simulink model "V2x_TC_CarBreakdownWarning_cs"  (Simulink 7.6)
settings: Solver=ode5  SolverMode=SingleTasking  StartTime=0.0  StopTime=18  FixedStep=1/100  RelTol=1e-3
PreLoadFcn:
  | check_NUTS_defined;
  | 
  | assignin('base',['model_closed_' bdroot],false);addpath('../includes_V2x');
InitFcn:
  | PreScanExperimentInitFcn(bdroot)
StopFcn:
  | PreScanExperimentStopFcn(bdroot)
undefined symbols (not defined in the file or in its folder): acceleration, actorID, actorType, DiscIntNeverNeededParam, GPS_alt, GPS_lat, GPS_long, intmax, lightBarInUse, messageID, Newton, publicActorType, Raphson, rotZ, sigbuilder_block, sireneInUse, trafficLightPriority, turnAdvice, velocity, x_ini_VRML, y_ini_VRML, yawRate, z_ini_VRML
libraries: simulink x61, PreScanSimulinkLibrary x19, PreScanUsefulBlocks x7, simulink_extras x1
(part 8 of 10)

== system V2x_TC_CarBreakdownWarning_cs/BMW_X5_1/Trajectories/Traj2State1 ==
  Traj Org : Inport
  Offset : Inport  Port=2
  Add2 : Sum
  ApplyRotation : PreScanSimulinkLibrary/ApplyRotation  SystemSampleTime=-1
  ApplyRotation1 : PreScanSimulinkLibrary/ApplyRotation  SystemSampleTime=-1
  ApplyRotation2 : PreScanSimulinkLibrary/ApplyRotation  SystemSampleTime=-1
  Constant : Constant  Value=zeros(12,1)
  Mux : Mux  Inputs=6
  Mux1 : Mux  Inputs=2
  Mux{2,4..9} (7 alike) : Mux  Inputs=3
  Mux3 : Mux  Inputs=2
  Selector : Selector  InputPortWidth=6  IndexOptions=Index vector (dialog)  Indices=[4 5 6]  OutputSizes=1
  Selector1 : Selector  InputPortWidth=21  IndexOptions=Index vector (dialog)  Indices=[5]  OutputSizes=1
  Selector10 : Selector  InputPortWidth=21  IndexOptions=Index vector (dialog)  Indices=[2]  OutputSizes=1
  Selector11 : Selector  InputPortWidth=21  IndexOptions=Index vector (dialog)  Indices=[3]  OutputSizes=1
  Selector12 : Selector  InputPortWidth=21  IndexOptions=Index vector (dialog)  Indices=[1]  OutputSizes=1
  Selector13 : Selector  InputPortWidth=21  IndexOptions=Index vector (dialog)  Indices=[8]  OutputSizes=1
  Selector14 : Selector  InputPortWidth=21  IndexOptions=Index vector (dialog)  Indices=[9]  OutputSizes=1
  Selector15 : Selector  InputPortWidth=21  IndexOptions=Index vector (dialog)  Indices=[7]  OutputSizes=1
  Selector16 : Selector  InputPortWidth=21  IndexOptions=Index vector (dialog)  Indices=[14]  OutputSizes=1
  Selector17 : Selector  InputPortWidth=21  IndexOptions=Index vector (dialog)  Indices=[15]  OutputSizes=1
  Selector18 : Selector  InputPortWidth=21  IndexOptions=Index vector (dialog)  Indices=[13]  OutputSizes=1
  Selector19 : Selector  InputPortWidth=21  IndexOptions=Index vector (dialog)  Indices=[20]  OutputSizes=1
  Selector2 : Selector  InputPortWidth=21  IndexOptions=Index vector (dialog)  Indices=[6]  OutputSizes=1
  Selector20 : Selector  InputPortWidth=21  IndexOptions=Index vector (dialog)  Indices=[21]  OutputSizes=1
  Selector21 : Selector  InputPortWidth=21  IndexOptions=Index vector (dialog)  Indices=[19]  OutputSizes=1
  Selector3 : Selector  InputPortWidth=21  IndexOptions=Index vector (dialog)  Indices=[12]  OutputSizes=1
  Selector4 : Selector  InputPortWidth=21  IndexOptions=Index vector (dialog)  Indices=[17]  OutputSizes=1
  Selector5 : Selector  InputPortWidth=21  IndexOptions=Index vector (dialog)  Indices=[18]  OutputSizes=1
  Selector6 : Selector  InputPortWidth=21  IndexOptions=Index vector (dialog)  Indices=[16]  OutputSizes=1
  Selector7 : Selector  InputPortWidth=21  IndexOptions=Index vector (dialog)  Indices=[11]  OutputSizes=1
  Selector8 : Selector  InputPortWidth=21  IndexOptions=Index vector (dialog)  Indices=[10]  OutputSizes=1
  Selector9 : Selector  InputPortWidth=21  IndexOptions=Index vector (dialog)  Indices=[4]  OutputSizes=1
  Traj2State2 : Subsystem
  state : Outport
  wires:
  Mux9/1 -> ApplyRotation2/2, ApplyRotation1/2, ApplyRotation/2
  Selector20/1 -> Mux9/3
  Selector19/1 -> Mux9/2
  Selector21/1 -> Mux9/1
  Selector5/1 -> Mux8/3
  Selector4/1 -> Mux8/2
  Selector6/1 -> Mux8/1
  Mux8/1 -> Mux/6
  Mux6/1 -> ApplyRotation2/1
  Mux7/1 -> Mux/4
  ApplyRotation2/1 -> Mux/5
  Selector3/1 -> Mux7/3
  Selector7/1 -> Mux7/2
  Selector8/1 -> Mux7/1
  Mux4/1 -> Mux/2
  Mux5/1 -> ApplyRotation1/1
  ApplyRotation1/1 -> Mux/3
  Mux2/1 -> ApplyRotation/1
  ApplyRotation/1 -> Mux/1
  Selector2/1 -> Mux4/3
  Selector1/1 -> Mux4/2
  Selector9/1 -> Mux4/1
  Selector17/1 -> Mux6/3
  Selector16/1 -> Mux6/2
  Selector18/1 -> Mux6/1
  Selector14/1 -> Mux5/3
  Selector13/1 -> Mux5/2
  Selector15/1 -> Mux5/1
  Selector11/1 -> Mux2/3
  Selector10/1 -> Mux2/2
  Selector12/1 -> Mux2/1
  Mux3/1 -> Selector8/1, Selector7/1, Selector3/1, Selector18/1, Selector16/1, Selector17/1, Selector6/1, Selector20/1, Selector19/1, Selector21/1, Selector5/1, Selector4/1, Selector14/1, Selector13/1, Selector15/1, Selector2/1, Selector1/1, Selector9/1, Selector12/1, Selector10/1, Selector11/1
  Mux1/1 -> Add2/2
  Constant/1 -> Mux1/2
  Add2/1 -> Traj2State2/1(traj)
  Selector/1 -> Mux3/2
  Traj Org/1 -> Mux3/1
  Offset/1 -> Mux1/1, Selector/1
  Mux/1 -> Add2/1
  Traj2State2/1(state) -> state/1

== system V2x_TC_CarBreakdownWarning_cs/BMW_X5_1/Trajectories/Trajectory_4 ==
  From Workspace : FromWorkspace  VariableName=trajectory  SampleTime=TimeStep  OutputAfterFinalValue=Holding final value
  From Workspace1 : FromWorkspace  VariableName=trajectory  SampleTime=TimeStep  OutputAfterFinalValue=Setting to zero
  Mux : Mux  Inputs=2
  Selector1 : Selector  InputPortWidth=24  IndexOptions=Index vector (dialog)  Indices=[7:18]  OutputSizes=1
  Selector9 : Selector  InputPortWidth=24  IndexOptions=Index vector (dialog)  Indices=[1:6]  OutputSizes=1
  trajectory : Outport
  wires:
  Selector1/1 -> Mux/2
  Selector9/1 -> Mux/1
  Mux/1 -> trajectory/1
  From Workspace1/1 -> Selector1/1
  From Workspace/1 -> Selector9/1

== system V2x_TC_CarBreakdownWarning_cs/BMW_X5_1/vehicle CAM generator/CAM generation ==
  x [m] : Inport
  y [m] : Inport  Port=2
  z [m] : Inport  Port=3
  rotZ [deg] : Inport  Port=4
  velocity [m/s] : Inport  Port=5
  Enable : EnablePort  StatesWhenEnabling=reset  PropagateVarSize=During execution
  Add : Sum  Inputs=+-
  Data Store Memory : DataStoreMemory  DataStoreName=CAM_time
  Data Store Memory1 : DataStoreMemory  DataStoreName=CAM_velocity
  Data Store Memory2 : DataStoreMemory  DataStoreName=CAM_heading
  Data Store Memory3 : DataStoreMemory  DataStoreName=CAM_x
  Data Store Memory4 : DataStoreMemory  DataStoreName=CAM_y
  Data Store Memory5 : DataStoreMemory  DataStoreName=CAM_z
  Data Store Read : DataStoreRead  DataStoreName=CAM_time  SampleTime=0.01
  Digital Clock : DigitalClock  SampleTime=0.01
  Merge : Merge  Inputs=3
  if : If  IfExpression=u1 >= 1  ElseIfExpressions=u1 < 0.1
  maybe : Subsystem  TreatAsAtomicUnit=on
  no : Subsystem  TreatAsAtomicUnit=on
  yes : Subsystem  TreatAsAtomicUnit=on
  CAN generation signal : Outport  OutputWhenDisabled=reset  InitialOutput=0
  wires:
  Digital Clock/1 -> Add/1
  Data Store Read/1 -> Add/2
  Add/1 -> if/1
  if/1 -> yes/Action
  yes/1(Out1) -> Merge/1
  no/1(Out1) -> Merge/2
  if/2 -> no/Action
  if/3 -> maybe/Action
  Merge/1 -> CAN generation signal/1
  x [m]/1 -> maybe/1(x [m]), yes/1(x [m])
  y [m]/1 -> maybe/2(y [m]), yes/2(y [m])
  z [m]/1 -> maybe/3(z [m]), yes/3(z [m])
  rotZ [deg]/1 -> maybe/4(rotZ [deg]), yes/4(rotZ [deg])
  velocity [m/s]/1 -> maybe/5(velocity [m/s]), yes/5(velocity [m/s])
  maybe/1(Out1) -> Merge/3

== system V2x_TC_CarBreakdownWarning_cs/BMW_X5_1/vehicle CAM generator/Enabled Subsystem ==
  CAM_sig : Inport
  Enable : EnablePort  PropagateVarSize=During execution
  CAM_signals : Outport  OutputWhenDisabled=reset  InitialOutput=0
  wires:
  CAM_sig/1 -> CAM_signals/1

== system V2x_TC_CarBreakdownWarning_cs/BMW_X5_1/vehicle CAM generator/impulse generator ==
  CAM_time_step : Inport
  Add : Sum
  Compare To Zero : simulink/Logic and Bit Operations/Compare To Zero  SystemSampleTime=-1  relop=>  LogicOutDataTypeMode=uint8  ZeroCross=off
  Data Type Conversion : DataTypeConversion  OutDataTypeStr=boolean
  Detect Change : simulink/Logic and Bit Operations/Detect Change  SystemSampleTime=-1  vinit=0
  Digital Clock1 : DigitalClock  SampleTime=0.01
  Divide : Product  Inputs=*/
  Gain : Gain  Gain=pi
  Product : Product  RndMeth=Zero
  Trigonometric Function : Trigonometry
  constant : Constant
  experiment time step : Constant  Value=0.01  SampleTime=0
  enable : Outport
  wires:
  Digital Clock1/1 -> Product/1
  Gain/1 -> Product/2
  Trigonometric Function/1 -> Compare To Zero/1
  Compare To Zero/1 -> Detect Change/1
  Detect Change/1 -> Data Type Conversion/1
  Product/1 -> Add/1
  constant/1 -> Divide/1
  Divide/1 -> Gain/1
  Add/1 -> Trigonometric Function/1
  experiment time step/1 -> Add/2
  Data Type Conversion/1 -> enable/1
  CAM_time_step/1 -> Divide/2

== system V2x_TC_CarBreakdownWarning_cs/BMW_X5_1/vehicle CAM generator/impulse generator1 ==
  CAM_time_step : Inport
  Add : Sum
  Compare To Zero : simulink/Logic and Bit Operations/Compare To Zero  SystemSampleTime=-1  relop=>  LogicOutDataTypeMode=uint8  ZeroCross=off
  Data Type Conversion : DataTypeConversion  OutDataTypeStr=boolean
  Detect Change : simulink/Logic and Bit Operations/Detect Change  SystemSampleTime=-1  vinit=0
  Digital Clock1 : DigitalClock  SampleTime=0.01
  Divide : Product  Inputs=*/
  Gain : Gain  Gain=pi
  Product : Product  RndMeth=Zero
  Trigonometric Function : Trigonometry
  constant : Constant
  experiment time step : Constant  Value=0.01  SampleTime=0
  enable : Outport
  wires:
  CAM_time_step/1 -> Divide/2
  Data Type Conversion/1 -> enable/1
  experiment time step/1 -> Add/2
  Add/1 -> Trigonometric Function/1
  Divide/1 -> Gain/1
  constant/1 -> Divide/1
  Product/1 -> Add/1
  Detect Change/1 -> Data Type Conversion/1
  Compare To Zero/1 -> Detect Change/1
  Trigonometric Function/1 -> Compare To Zero/1
  Gain/1 -> Product/2
  Digital Clock1/1 -> Product/1

== system V2x_TC_CarBreakdownWarning_cs/BMW_X5_1/vehicle CAM generator/set CAM signals ==
  CAM generation signal : Inport
  warning : Inport  Port=2
  messageID : Inport  Port=3
  actorID : Inport  Port=4
  actorType : Inport  Port=5
  publicActorType : Inport  Port=6
  lightBarInUse : Inport  Port=7
  sireneInUse : Inport  Port=8
  velocity : Inport  Port=9
  acceleration : Inport  Port=10
  yawRate : Inport  Port=11
  turnAdvice : Inport  Port=12
  trafficLightPriority : Inport  Port=13
  GPS_lat : Inport  Port=14
  GPS_long : Inport  Port=15
  GPS_alt : Inport  Port=16
  rotZ : Inport  Port=17
  Mux : Mux  Inputs=16
  Switch : Switch  Criteria=u2 > Threshold  Threshold=0.5
  Unit Delay : UnitDelay  SampleTime=-1
  CAM_signals : Outport
  wires:
  warning/1 -> Mux/1
  messageID/1 -> Mux/2
  actorID/1 -> Mux/3
  actorType/1 -> Mux/4
  publicActorType/1 -> Mux/5
  lightBarInUse/1 -> Mux/6
  sireneInUse/1 -> Mux/7
  velocity/1 -> Mux/8
  acceleration/1 -> Mux/9
  yawRate/1 -> Mux/10
  turnAdvice/1 -> Mux/11
  trafficLightPriority/1 -> Mux/12
  GPS_lat/1 -> Mux/13
  GPS_long/1 -> Mux/14
  GPS_alt/1 -> Mux/15
  rotZ/1 -> Mux/16
  CAM generation signal/1 -> Switch/2
  Mux/1 -> Switch/1
  Switch/1 -> Unit Delay/1, CAM_signals/1
  Unit Delay/1 -> Switch/3

== system V2x_TC_CarBreakdownWarning_cs/CameraTrolley/Dynamics_Empty/MuxState ==
  note: mode: Dynamics
  note: mode: Positioning
  note: mode: Dynamics
      | VelVEHICLE
      | wrt VEH
  note: AnglesVEHICLE
      | wrtGLOB
  note: For state mode 'Dynamic' positions
      | are not taken into account, as they
      | are computed by integrating velocity.
      | Click annotation for Help.
  x [m] : Inport  SampleTime=TimeStep
  y [m] : Inport  Port=2  SampleTime=TimeStep
  z [m] : Inport  Port=3  SampleTime=TimeStep
  dx [m/s] : Inport  Port=4  SampleTime=TimeStep
  dy [m/s] : Inport  Port=5  SampleTime=TimeStep
  dz [m/s] : Inport  Port=6  SampleTime=TimeStep
  R [rad] : Inport  Port=7  SampleTime=TimeStep
  P [rad] : Inport  Port=8  SampleTime=TimeStep
  Y [rad] : Inport  Port=9  SampleTime=TimeStep
  Constant : Constant  DisableCoverage=on  Value=positioningmode
  Discrete-Time Integrator : DiscreteIntegrator  SampleTime=TimeStep  ICPrevOutput=DiscIntNeverNeededParam  ICPrevScaledInput=DiscIntNeverNeededParam
  Ground : Ground
  Ground1 : Ground
  Mux1 : Mux  Inputs=[3 3]
  Mux2 : Mux  Inputs=3
  Mux3 : Mux  Inputs=3
  Mux4 : Mux  Inputs=3
  Mux5 : Mux  Inputs=[3 3]
  Mux6 : Mux  Inputs=[6 3]
  Switch : Switch  Threshold=0.5
  Transformation_BODY2GLOBAL : PreScanSimulinkLibrary/Simple_Vehicle_Dynamics/Chassis/MuxDynState/Transformation_BODY2GLOBAL  SystemSampleTime=-1
  mux3 : Mux  Inputs=3
  state : Outport
  wires:
  Constant/1 -> Switch/2
  Mux6/1 -> state/1
  Mux4/1 -> Mux1/1
  Mux5/1 -> Switch/3
  Mux1/1 -> Switch/1
  Switch/1 -> Mux6/1  "PosVeh wrt  GLOB"
  P [rad]/1 -> Mux3/2
  R [rad]/1 -> Mux3/1
  dz [m/s]/1 -> Mux2/3
  dy [m/s]/1 -> Mux2/2
  dx [m/s]/1 -> Mux2/1
  z [m]/1 -> Mux4/3
  y [m]/1 -> Mux4/2
  x [m]/1 -> Mux4/1
  Ground1/1 -> mux3/2  "pitch"
  Y [rad]/1 -> mux3/3, Mux3/3  "yaw"
  Mux3/1 -> Mux6/2
  Transformation_BODY2GLOBAL/1 -> Discrete-Time Integrator/1, Mux5/2  "VelVEH wrt  GLOB"
  mux3/1 -> Transformation_BODY2GLOBAL/2
  Ground/1 -> mux3/1  "roll"
  Mux2/1 -> Mux1/2, Transformation_BODY2GLOBAL/1
  Discrete-Time Integrator/1 -> Mux5/1  "PosVEH wrt  GLOB"

== system V2x_TC_CarBreakdownWarning_cs/CameraTrolley/SELF_Demux/compas converter ==
  rotz [rad] : Inport
  cart2compas : Subsystem
  rad2deg : Gain  Gain=180/pi
  heading [deg] : Outport
  wires:
  cart2compas/1(heading [deg]) -> heading [deg]/1
  rotz [rad]/1 -> rad2deg/1
  rad2deg/1 -> cart2compas/1(Angle [deg])

== system V2x_TC_CarBreakdownWarning_cs/Fiat_Bravo_1/SELF_Demux/compas converter ==
  rotz [rad] : Inport
  cart2compas : Subsystem
  rad2deg : Gain  Gain=180/pi
  heading [deg] : Outport
  wires:
  cart2compas/1(heading [deg]) -> heading [deg]/1
  rotz [rad]/1 -> rad2deg/1
  rad2deg/1 -> cart2compas/1(Angle [deg])

== system V2x_TC_CarBreakdownWarning_cs/Fiat_Bravo_1/Trajectories/Traj2State1 ==
  Traj Org : Inport
  Offset : Inport  Port=2
  Add2 : Sum
  ApplyRotation : PreScanSimulinkLibrary/ApplyRotation  SystemSampleTime=-1
  ApplyRotation1 : PreScanSimulinkLibrary/ApplyRotation  SystemSampleTime=-1
  ApplyRotation2 : PreScanSimulinkLibrary/ApplyRotation  SystemSampleTime=-1
  Constant : Constant  Value=zeros(12,1)
  Mux : Mux  Inputs=6
  Mux1 : Mux  Inputs=2
  Mux{2,4..9} (7 alike) : Mux  Inputs=3
  Mux3 : Mux  Inputs=2
  Selector : Selector  InputPortWidth=6  IndexOptions=Index vector (dialog)  Indices=[4 5 6]  OutputSizes=1
  Selector1 : Selector  InputPortWidth=21  IndexOptions=Index vector (dialog)  Indices=[5]  OutputSizes=1
  Selector10 : Selector  InputPortWidth=21  IndexOptions=Index vector (dialog)  Indices=[2]  OutputSizes=1
  Selector11 : Selector  InputPortWidth=21  IndexOptions=Index vector (dialog)  Indices=[3]  OutputSizes=1
  Selector12 : Selector  InputPortWidth=21  IndexOptions=Index vector (dialog)  Indices=[1]  OutputSizes=1
  Selector13 : Selector  InputPortWidth=21  IndexOptions=Index vector (dialog)  Indices=[8]  OutputSizes=1
  Selector14 : Selector  InputPortWidth=21  IndexOptions=Index vector (dialog)  Indices=[9]  OutputSizes=1
  Selector15 : Selector  InputPortWidth=21  IndexOptions=Index vector (dialog)  Indices=[7]  OutputSizes=1
  Selector16 : Selector  InputPortWidth=21  IndexOptions=Index vector (dialog)  Indices=[14]  OutputSizes=1
  Selector17 : Selector  InputPortWidth=21  IndexOptions=Index vector (dialog)  Indices=[15]  OutputSizes=1
  Selector18 : Selector  InputPortWidth=21  IndexOptions=Index vector (dialog)  Indices=[13]  OutputSizes=1
  Selector19 : Selector  InputPortWidth=21  IndexOptions=Index vector (dialog)  Indices=[20]  OutputSizes=1
  Selector2 : Selector  InputPortWidth=21  IndexOptions=Index vector (dialog)  Indices=[6]  OutputSizes=1
  Selector20 : Selector  InputPortWidth=21  IndexOptions=Index vector (dialog)  Indices=[21]  OutputSizes=1
  Selector21 : Selector  InputPortWidth=21  IndexOptions=Index vector (dialog)  Indices=[19]  OutputSizes=1
  Selector3 : Selector  InputPortWidth=21  IndexOptions=Index vector (dialog)  Indices=[12]  OutputSizes=1
  Selector4 : Selector  InputPortWidth=21  IndexOptions=Index vector (dialog)  Indices=[17]  OutputSizes=1
  Selector5 : Selector  InputPortWidth=21  IndexOptions=Index vector (dialog)  Indices=[18]  OutputSizes=1
  Selector6 : Selector  InputPortWidth=21  IndexOptions=Index vector (dialog)  Indices=[16]  OutputSizes=1
  Selector7 : Selector  InputPortWidth=21  IndexOptions=Index vector (dialog)  Indices=[11]  OutputSizes=1
  Selector8 : Selector  InputPortWidth=21  IndexOptions=Index vector (dialog)  Indices=[10]  OutputSizes=1
  Selector9 : Selector  InputPortWidth=21  IndexOptions=Index vector (dialog)  Indices=[4]  OutputSizes=1
  Traj2State2 : Subsystem
  state : Outport
  wires:
  Mux9/1 -> ApplyRotation2/2, ApplyRotation1/2, ApplyRotation/2
  Selector20/1 -> Mux9/3
  Selector19/1 -> Mux9/2
  Selector21/1 -> Mux9/1
  Selector5/1 -> Mux8/3
  Selector4/1 -> Mux8/2
  Selector6/1 -> Mux8/1
  Mux8/1 -> Mux/6
  Mux6/1 -> ApplyRotation2/1
  Mux7/1 -> Mux/4
  ApplyRotation2/1 -> Mux/5
  Selector3/1 -> Mux7/3
  Selector7/1 -> Mux7/2
  Selector8/1 -> Mux7/1
  Mux4/1 -> Mux/2
  Mux5/1 -> ApplyRotation1/1
  ApplyRotation1/1 -> Mux/3
  Mux2/1 -> ApplyRotation/1
  ApplyRotation/1 -> Mux/1
  Selector2/1 -> Mux4/3
  Selector1/1 -> Mux4/2
  Selector9/1 -> Mux4/1
  Selector17/1 -> Mux6/3
  Selector16/1 -> Mux6/2
  Selector18/1 -> Mux6/1
  Selector14/1 -> Mux5/3
  Selector13/1 -> Mux5/2
  Selector15/1 -> Mux5/1
  Selector11/1 -> Mux2/3
  Selector10/1 -> Mux2/2
  Selector12/1 -> Mux2/1
  Mux3/1 -> Selector8/1, Selector7/1, Selector3/1, Selector18/1, Selector16/1, Selector17/1, Selector6/1, Selector20/1, Selector19/1, Selector21/1, Selector5/1, Selector4/1, Selector14/1, Selector13/1, Selector15/1, Selector2/1, Selector1/1, Selector9/1, Selector12/1, Selector10/1, Selector11/1
  Mux1/1 -> Add2/2
  Constant/1 -> Mux1/2
  Add2/1 -> Traj2State2/1(traj)
  Selector/1 -> Mux3/2
  Traj Org/1 -> Mux3/1
  Offset/1 -> Mux1/1, Selector/1
  Mux/1 -> Add2/1
  Traj2State2/1(state) -> state/1

== system V2x_TC_CarBreakdownWarning_cs/Fiat_Bravo_1/Trajectories/Trajectory_3 ==
  From Workspace : FromWorkspace  VariableName=trajectory  SampleTime=TimeStep  OutputAfterFinalValue=Holding final value
  From Workspace1 : FromWorkspace  VariableName=trajectory  SampleTime=TimeStep  OutputAfterFinalValue=Setting to zero
  Mux : Mux  Inputs=2
  Selector1 : Selector  InputPortWidth=24  IndexOptions=Index vector (dialog)  Indices=[7:18]  OutputSizes=1
  Selector9 : Selector  InputPortWidth=24  IndexOptions=Index vector (dialog)  Indices=[1:6]  OutputSizes=1
  trajectory : Outport
  wires:
  Selector1/1 -> Mux/2
  Selector9/1 -> Mux/1
  Mux/1 -> trajectory/1
  From Workspace1/1 -> Selector1/1
  From Workspace/1 -> Selector9/1

== system V2x_TC_CarBreakdownWarning_cs/Fiat_Bravo_1/vehicle CAM generator/CAM generation ==
  x [m] : Inport
  y [m] : Inport  Port=2
  z [m] : Inport  Port=3
  rotZ [deg] : Inport  Port=4
  velocity [m/s] : Inport  Port=5
  Enable : EnablePort  StatesWhenEnabling=reset  PropagateVarSize=During execution
  Add : Sum  Inputs=+-
  Data Store Memory : DataStoreMemory  DataStoreName=CAM_time
  Data Store Memory1 : DataStoreMemory  DataStoreName=CAM_velocity
  Data Store Memory2 : DataStoreMemory  DataStoreName=CAM_heading
  Data Store Memory3 : DataStoreMemory  DataStoreName=CAM_x
  Data Store Memory4 : DataStoreMemory  DataStoreName=CAM_y
  Data Store Memory5 : DataStoreMemory  DataStoreName=CAM_z
  Data Store Read : DataStoreRead  DataStoreName=CAM_time  SampleTime=0.01
  Digital Clock : DigitalClock  SampleTime=0.01
  Merge : Merge  Inputs=3
  if : If  IfExpression=u1 >= 1  ElseIfExpressions=u1 < 0.1
  maybe : Subsystem  TreatAsAtomicUnit=on
  no : Subsystem  TreatAsAtomicUnit=on
  yes : Subsystem  TreatAsAtomicUnit=on
  CAN generation signal : Outport  OutputWhenDisabled=reset  InitialOutput=0
  wires:
  Digital Clock/1 -> Add/1
  Data Store Read/1 -> Add/2
  Add/1 -> if/1
  if/1 -> yes/Action
  yes/1(Out1) -> Merge/1
  no/1(Out1) -> Merge/2
  if/2 -> no/Action
  if/3 -> maybe/Action
  Merge/1 -> CAN generation signal/1
  x [m]/1 -> maybe/1(x [m]), yes/1(x [m])
  y [m]/1 -> maybe/2(y [m]), yes/2(y [m])
  z [m]/1 -> maybe/3(z [m]), yes/3(z [m])
  rotZ [deg]/1 -> maybe/4(rotZ [deg]), yes/4(rotZ [deg])
  velocity [m/s]/1 -> maybe/5(velocity [m/s]), yes/5(velocity [m/s])
  maybe/1(Out1) -> Merge/3

== system V2x_TC_CarBreakdownWarning_cs/Fiat_Bravo_1/vehicle CAM generator/Enabled Subsystem ==
  CAM_sig : Inport
  Enable : EnablePort  PropagateVarSize=During execution
  CAM_signals : Outport  OutputWhenDisabled=reset  InitialOutput=0
  wires:
  CAM_sig/1 -> CAM_signals/1

== system V2x_TC_CarBreakdownWarning_cs/Fiat_Bravo_1/vehicle CAM generator/impulse generator ==
  CAM_time_step : Inport
  Add : Sum
  Compare To Zero : simulink/Logic and Bit Operations/Compare To Zero  SystemSampleTime=-1  relop=>  LogicOutDataTypeMode=uint8  ZeroCross=off
  Data Type Conversion : DataTypeConversion  OutDataTypeStr=boolean
  Detect Change : simulink/Logic and Bit Operations/Detect Change  SystemSampleTime=-1  vinit=0
  Digital Clock1 : DigitalClock  SampleTime=0.01
  Divide : Product  Inputs=*/
  Gain : Gain  Gain=pi
  Product : Product  RndMeth=Zero
  Trigonometric Function : Trigonometry
  constant : Constant
  experiment time step : Constant  Value=0.01  SampleTime=0
  enable : Outport
  wires:
  Digital Clock1/1 -> Product/1
  Gain/1 -> Product/2
  Trigonometric Function/1 -> Compare To Zero/1
  Compare To Zero/1 -> Detect Change/1
  Detect Change/1 -> Data Type Conversion/1
  Product/1 -> Add/1
  constant/1 -> Divide/1
  Divide/1 -> Gain/1
  Add/1 -> Trigonometric Function/1
  experiment time step/1 -> Add/2
  Data Type Conversion/1 -> enable/1
  CAM_time_step/1 -> Divide/2

== system V2x_TC_CarBreakdownWarning_cs/Fiat_Bravo_1/vehicle CAM generator/impulse generator1 ==
  CAM_time_step : Inport
  Add : Sum
  Compare To Zero : simulink/Logic and Bit Operations/Compare To Zero  SystemSampleTime=-1  relop=>  LogicOutDataTypeMode=uint8  ZeroCross=off
  Data Type Conversion : DataTypeConversion  OutDataTypeStr=boolean
  Detect Change : simulink/Logic and Bit Operations/Detect Change  SystemSampleTime=-1  vinit=0
  Digital Clock1 : DigitalClock  SampleTime=0.01
  Divide : Product  Inputs=*/
  Gain : Gain  Gain=pi
  Product : Product  RndMeth=Zero
  Trigonometric Function : Trigonometry
  constant : Constant
  experiment time step : Constant  Value=0.01  SampleTime=0
  enable : Outport
  wires:
  CAM_time_step/1 -> Divide/2
  Data Type Conversion/1 -> enable/1
  experiment time step/1 -> Add/2
  Add/1 -> Trigonometric Function/1
  Divide/1 -> Gain/1
  constant/1 -> Divide/1
  Product/1 -> Add/1
  Detect Change/1 -> Data Type Conversion/1
  Compare To Zero/1 -> Detect Change/1
  Trigonometric Function/1 -> Compare To Zero/1
  Gain/1 -> Product/2
  Digital Clock1/1 -> Product/1

== system V2x_TC_CarBreakdownWarning_cs/Fiat_Bravo_1/vehicle CAM generator/set CAM signals ==
  CAM generation signal : Inport
  warning : Inport  Port=2
  messageID : Inport  Port=3
  actorID : Inport  Port=4
  actorType : Inport  Port=5
  publicActorType : Inport  Port=6
  lightBarInUse : Inport  Port=7
  sireneInUse : Inport  Port=8
  velocity : Inport  Port=9
  acceleration : Inport  Port=10
  yawRate : Inport  Port=11
  turnAdvice : Inport  Port=12
  trafficLightPriority : Inport  Port=13
  GPS_lat : Inport  Port=14
  GPS_long : Inport  Port=15
  GPS_alt : Inport  Port=16
  rotZ : Inport  Port=17
  Mux : Mux  Inputs=16
  Switch : Switch  Criteria=u2 > Threshold  Threshold=0.5
  Unit Delay : UnitDelay  SampleTime=-1
  CAM_signals : Outport
  wires:
  warning/1 -> Mux/1
  messageID/1 -> Mux/2
  actorID/1 -> Mux/3
  actorType/1 -> Mux/4
  publicActorType/1 -> Mux/5
  lightBarInUse/1 -> Mux/6
  sireneInUse/1 -> Mux/7
  velocity/1 -> Mux/8
  acceleration/1 -> Mux/9
  yawRate/1 -> Mux/10
  turnAdvice/1 -> Mux/11
  trafficLightPriority/1 -> Mux/12
  GPS_lat/1 -> Mux/13
  GPS_long/1 -> Mux/14
  GPS_alt/1 -> Mux/15
  rotZ/1 -> Mux/16
  CAM generation signal/1 -> Switch/2
  Mux/1 -> Switch/1
  Switch/1 -> Unit Delay/1, CAM_signals/1
  Unit Delay/1 -> Switch/3

== system V2x_TC_CarBreakdownWarning_cs/Toyota_Previa_1/Antenna_Rx_1_Demux/Reorder ==
  In : Inport
  Selector1 : Selector  InputPortWidth=InputPortWidth  IndexOptions=Index vector (dialog)  Indices=Elements  OutputSizes=1
  Out : Outport
  wires:
  Selector1/1 -> Out/1
  In/1 -> Selector1/1

== system V2x_TC_CarBreakdownWarning_cs/Toyota_Previa_1/Antenna_Rx_1_Demux/compas converter ==
  rotz [rad] : Inport
  cart2compas : Subsystem
  rad2deg : Gain  Gain=180/pi
  heading [deg] : Outport
  wires:
  rad2deg/1 -> cart2compas/1(Angle [deg])
  rotz [rad]/1 -> rad2deg/1
  cart2compas/1(heading [deg]) -> heading [deg]/1

== system V2x_TC_CarBreakdownWarning_cs/Toyota_Previa_1/Dynamics_Empty/MuxState ==
  note: mode: Dynamics
  note: mode: Positioning
  note: mode: Dynamics
      | VelVEHICLE
      | wrt VEH
  note: AnglesVEHICLE
      | wrtGLOB
  note: For state mode 'Dynamic' positions
      | are not taken into account, as they
      | are computed by integrating velocity.
      | Click annotation for Help.
  x [m] : Inport  SampleTime=TimeStep
  y [m] : Inport  Port=2  SampleTime=TimeStep
  z [m] : Inport  Port=3  SampleTime=TimeStep
  dx [m/s] : Inport  Port=4  SampleTime=TimeStep
  dy [m/s] : Inport  Port=5  SampleTime=TimeStep
  dz [m/s] : Inport  Port=6  SampleTime=TimeStep
  R [rad] : Inport  Port=7  SampleTime=TimeStep
  P [rad] : Inport  Port=8  SampleTime=TimeStep
  Y [rad] : Inport  Port=9  SampleTime=TimeStep
  Constant : Constant  DisableCoverage=on  Value=positioningmode
  Discrete-Time Integrator : DiscreteIntegrator  SampleTime=TimeStep  ICPrevOutput=DiscIntNeverNeededParam  ICPrevScaledInput=DiscIntNeverNeededParam
  Ground : Ground
  Ground1 : Ground
  Mux1 : Mux  Inputs=[3 3]
  Mux2 : Mux  Inputs=3
  Mux3 : Mux  Inputs=3
  Mux4 : Mux  Inputs=3
  Mux5 : Mux  Inputs=[3 3]
  Mux6 : Mux  Inputs=[6 3]
  Switch : Switch  Threshold=0.5
  Transformation_BODY2GLOBAL : PreScanSimulinkLibrary/Simple_Vehicle_Dynamics/Chassis/MuxDynState/Transformation_BODY2GLOBAL  SystemSampleTime=-1
  mux3 : Mux  Inputs=3
  state : Outport
  wires:
  Constant/1 -> Switch/2
  Mux6/1 -> state/1
  Mux4/1 -> Mux1/1
  Mux5/1 -> Switch/3
  Mux1/1 -> Switch/1
  Switch/1 -> Mux6/1  "PosVeh wrt  GLOB"
  P [rad]/1 -> Mux3/2
  R [rad]/1 -> Mux3/1
  dz [m/s]/1 -> Mux2/3
  dy [m/s]/1 -> Mux2/2
  dx [m/s]/1 -> Mux2/1
  z [m]/1 -> Mux4/3
  y [m]/1 -> Mux4/2
  x [m]/1 -> Mux4/1
  Ground1/1 -> mux3/2  "pitch"
  Y [rad]/1 -> mux3/3, Mux3/3  "yaw"
  Mux3/1 -> Mux6/2
  Transformation_BODY2GLOBAL/1 -> Discrete-Time Integrator/1, Mux5/2  "VelVEH wrt  GLOB"
  mux3/1 -> Transformation_BODY2GLOBAL/2
  Ground/1 -> mux3/1  "roll"
  Mux2/1 -> Mux1/2, Transformation_BODY2GLOBAL/1
  Discrete-Time Integrator/1 -> Mux5/1  "PosVEH wrt  GLOB"

== system V2x_TC_CarBreakdownWarning_cs/Toyota_Previa_1/SELF_Demux/compas converter ==
  rotz [rad] : Inport
  cart2compas : Subsystem
  rad2deg : Gain  Gain=180/pi
  heading [deg] : Outport
  wires:
  cart2compas/1(heading [deg]) -> heading [deg]/1
  rotz [rad]/1 -> rad2deg/1
  rad2deg/1 -> cart2compas/1(Angle [deg])

== system V2x_TC_CarBreakdownWarning_cs/Toyota_Previa_1/vehicle CAM generator/CAM generation ==
  x [m] : Inport
  y [m] : Inport  Port=2
  z [m] : Inport  Port=3
  rotZ [deg] : Inport  Port=4
  velocity [m/s] : Inport  Port=5
  Enable : EnablePort  StatesWhenEnabling=reset  PropagateVarSize=During execution
  Add : Sum  Inputs=+-
  Data Store Memory : DataStoreMemory  DataStoreName=CAM_time
  Data Store Memory1 : DataStoreMemory  DataStoreName=CAM_velocity
  Data Store Memory2 : DataStoreMemory  DataStoreName=CAM_heading
  Data Store Memory3 : DataStoreMemory  DataStoreName=CAM_x
  Data Store Memory4 : DataStoreMemory  DataStoreName=CAM_y
  Data Store Memory5 : DataStoreMemory  DataStoreName=CAM_z
  Data Store Read : DataStoreRead  DataStoreName=CAM_time  SampleTime=0.01
  Digital Clock : DigitalClock  SampleTime=0.01
  Merge : Merge  Inputs=3
  if : If  IfExpression=u1 >= 1  ElseIfExpressions=u1 < 0.1
  maybe : Subsystem  TreatAsAtomicUnit=on
  no : Subsystem  TreatAsAtomicUnit=on
  yes : Subsystem  TreatAsAtomicUnit=on
  CAN generation signal : Outport  OutputWhenDisabled=reset  InitialOutput=0
  wires:
  Digital Clock/1 -> Add/1
  Data Store Read/1 -> Add/2
  Add/1 -> if/1
  if/1 -> yes/Action
  yes/1(Out1) -> Merge/1
  no/1(Out1) -> Merge/2
  if/2 -> no/Action
  if/3 -> maybe/Action
  Merge/1 -> CAN generation signal/1
  x [m]/1 -> maybe/1(x [m]), yes/1(x [m])
  y [m]/1 -> maybe/2(y [m]), yes/2(y [m])
  z [m]/1 -> maybe/3(z [m]), yes/3(z [m])
  rotZ [deg]/1 -> maybe/4(rotZ [deg]), yes/4(rotZ [deg])
  velocity [m/s]/1 -> maybe/5(velocity [m/s]), yes/5(velocity [m/s])
  maybe/1(Out1) -> Merge/3

== system V2x_TC_CarBreakdownWarning_cs/Toyota_Previa_1/vehicle CAM generator/Enabled Subsystem ==
  CAM_sig : Inport
  Enable : EnablePort  PropagateVarSize=During execution
  CAM_signals : Outport  OutputWhenDisabled=reset  InitialOutput=0
  wires:
  CAM_sig/1 -> CAM_signals/1

== system V2x_TC_CarBreakdownWarning_cs/Toyota_Previa_1/vehicle CAM generator/Subsystem ==
  In1 : Inport
  GPS_Noise_src : Inport  Port=2
  GPS Noise : Subsystem
  Sum2 : Sum  Inputs=|++
  Out1 : Outport
  wires:
  GPS Noise/1(GPS_Noise) -> Sum2/2
  In1/1 -> Sum2/1
  Sum2/1 -> Out1/1
  GPS_Noise_src/1 -> GPS Noise/1(GPS_Noise_src)

== system V2x_TC_CarBreakdownWarning_cs/Toyota_Previa_1/vehicle CAM generator/Subsystem1 ==
  In1 : Inport
  GPS_Noise_src : Inport  Port=2
  GPS Noise : Subsystem
  Sum2 : Sum  Inputs=|++
  Out1 : Outport
  wires:
  GPS_Noise_src/1 -> GPS Noise/1(GPS_Noise_src)
  Sum2/1 -> Out1/1
  In1/1 -> Sum2/1
  GPS Noise/1(GPS_Noise) -> Sum2/2

== system V2x_TC_CarBreakdownWarning_cs/Toyota_Previa_1/vehicle CAM generator/Subsystem2 ==
  In1 : Inport
  GPS_Noise_src : Inport  Port=2
  GPS Noise : Subsystem
  Sum2 : Sum  Inputs=|++
  Out1 : Outport
  wires:
  GPS Noise/1(GPS_Noise) -> Sum2/2
  In1/1 -> Sum2/1
  Sum2/1 -> Out1/1
  GPS_Noise_src/1 -> GPS Noise/1(GPS_Noise_src)

== system V2x_TC_CarBreakdownWarning_cs/Toyota_Previa_1/vehicle CAM generator/Subsystem3 ==
  In1 : Inport
  GPS_Noise_src : Inport  Port=2
  GPS Noise : Subsystem
  Sum2 : Sum  Inputs=|++
  Out1 : Outport
  wires:
  GPS_Noise_src/1 -> GPS Noise/1(GPS_Noise_src)
  Sum2/1 -> Out1/1
  In1/1 -> Sum2/1
  GPS Noise/1(GPS_Noise) -> Sum2/2

== system V2x_TC_CarBreakdownWarning_cs/Toyota_Previa_1/vehicle CAM generator/impulse generator ==
  CAM_time_step : Inport
  Add : Sum
  Compare To Zero : simulink/Logic and Bit Operations/Compare To Zero  SystemSampleTime=-1  relop=>  LogicOutDataTypeMode=uint8  ZeroCross=off
  Data Type Conversion : DataTypeConversion  OutDataTypeStr=boolean
  Detect Change : simulink/Logic and Bit Operations/Detect Change  SystemSampleTime=-1  vinit=0
  Digital Clock1 : DigitalClock  SampleTime=0.01
  Divide : Product  Inputs=*/
  Gain : Gain  Gain=pi
  Product : Product  RndMeth=Zero
  Trigonometric Function : Trigonometry
  constant : Constant
  experiment time step : Constant  Value=0.01  SampleTime=0
  enable : Outport
  wires:
  Digital Clock1/1 -> Product/1
  Gain/1 -> Product/2
  Trigonometric Function/1 -> Compare To Zero/1
  Compare To Zero/1 -> Detect Change/1
  Detect Change/1 -> Data Type Conversion/1
  Product/1 -> Add/1
  constant/1 -> Divide/1
  Divide/1 -> Gain/1
  Add/1 -> Trigonometric Function/1
  experiment time step/1 -> Add/2
  Data Type Conversion/1 -> enable/1
  CAM_time_step/1 -> Divide/2

== system V2x_TC_CarBreakdownWarning_cs/Toyota_Previa_1/vehicle CAM generator/impulse generator1 ==
  CAM_time_step : Inport
  Add : Sum
  Compare To Zero : simulink/Logic and Bit Operations/Compare To Zero  SystemSampleTime=-1  relop=>  LogicOutDataTypeMode=uint8  ZeroCross=off
  Data Type Conversion : DataTypeConversion  OutDataTypeStr=boolean
  Detect Change : simulink/Logic and Bit Operations/Detect Change  SystemSampleTime=-1  vinit=0
  Digital Clock1 : DigitalClock  SampleTime=0.01
  Divide : Product  Inputs=*/
  Gain : Gain  Gain=pi
  Product : Product  RndMeth=Zero
  Trigonometric Function : Trigonometry
  constant : Constant
  experiment time step : Constant  Value=0.01  SampleTime=0
  enable : Outport
  wires:
  CAM_time_step/1 -> Divide/2
  Data Type Conversion/1 -> enable/1
  experiment time step/1 -> Add/2
  Add/1 -> Trigonometric Function/1
  Divide/1 -> Gain/1
  constant/1 -> Divide/1
  Product/1 -> Add/1
  Detect Change/1 -> Data Type Conversion/1
  Compare To Zero/1 -> Detect Change/1
  Trigonometric Function/1 -> Compare To Zero/1
  Gain/1 -> Product/2
  Digital Clock1/1 -> Product/1

== system V2x_TC_CarBreakdownWarning_cs/Toyota_Previa_1/vehicle CAM generator/set CAM signals ==
  CAM generation signal : Inport
  warning : Inport  Port=2
  messageID : Inport  Port=3
  actorID : Inport  Port=4
  actorType : Inport  Port=5
  publicActorType : Inport  Port=6
  lightBarInUse : Inport  Port=7
  sireneInUse : Inport  Port=8
  velocity : Inport  Port=9
  acceleration : Inport  Port=10
  yawRate : Inport  Port=11
  turnAdvice : Inport  Port=12
  trafficLightPriority : Inport  Port=13
  GPS_lat : Inport  Port=14
  GPS_long : Inport  Port=15
  GPS_alt : Inport  Port=16
  rotZ : Inport  Port=17
  Mux : Mux  Inputs=16
  Switch : Switch  Criteria=u2 > Threshold  Threshold=0.5
  Unit Delay : UnitDelay  SampleTime=-1
  CAM_signals : Outport
  wires:
  warning/1 -> Mux/1
  messageID/1 -> Mux/2
  actorID/1 -> Mux/3
  actorType/1 -> Mux/4
  publicActorType/1 -> Mux/5
  lightBarInUse/1 -> Mux/6
  sireneInUse/1 -> Mux/7
  velocity/1 -> Mux/8
  acceleration/1 -> Mux/9
  yawRate/1 -> Mux/10
  turnAdvice/1 -> Mux/11
  trafficLightPriority/1 -> Mux/12
  GPS_lat/1 -> Mux/13
  GPS_long/1 -> Mux/14
  GPS_alt/1 -> Mux/15
  rotZ/1 -> Mux/16
  CAM generation signal/1 -> Switch/2
  Mux/1 -> Switch/1
  Switch/1 -> Unit Delay/1, CAM_signals/1
  Unit Delay/1 -> Switch/3

== system V2x_TC_CarBreakdownWarning_cs/VISUWheels_Audi_A8_1/conv_RotWheelFL/RotMat2AxisAngle ==
  RotMat_Visu : Inport
  Data Type Conversion : DataTypeConversion
  Divide : Product  Inputs=*/
  Gain : Gain  Gain=2
  Mux : Mux  Inputs=3
  Mux1 : Mux  Inputs=2
  Saturation1 : Saturate  UpperLimit=3-0.001  LowerLimit=-1+0.001
  Trigonometric Function : Trigonometry
  U1 : Fcn  Expr=u[6]-u[8]
  U2 : Fcn  Expr=u[7]-u[3]
  U3 : Fcn  Expr=u[2]-u[4]
  U_Phi : Fcn  Expr=u[1]+u[5]+u[9]
  U_Phi1 : Fcn  Expr=acos((u(1)-1)/2)
  U_Phi2 : Fcn  Expr=acos((u(1)-1)/2)
  Angles_Visu : Outport
  wires:
  U_Phi2/1 -> Trigonometric Function/1
  Saturation1/1 -> U_Phi2/1
  U_Phi1/1 -> Data Type Conversion/1
  U_Phi/1 -> Saturation1/1, U_Phi1/1
  Divide/1 -> Mux1/1
  Mux1/1 -> Angles_Visu/1
  Gain/1 -> Divide/2
  Mux/1 -> Divide/1
  U3/1 -> Mux/3
  U2/1 -> Mux/2
  U1/1 -> Mux/1
  Trigonometric Function/1 -> Gain/1
  RotMat_Visu/1 -> U_Phi/1, U3/1, U2/1, U1/1
  Data Type Conversion/1 -> Mux1/2

== system V2x_TC_CarBreakdownWarning_cs/VISUWheels_Audi_A8_1/conv_RotWheelFR/RotMat2AxisAngle ==
  RotMat_Visu : Inport
  Data Type Conversion : DataTypeConversion
  Divide : Product  Inputs=*/
  Gain : Gain  Gain=2
  Mux : Mux  Inputs=3
  Mux1 : Mux  Inputs=2
  Saturation1 : Saturate  UpperLimit=3-0.001  LowerLimit=-1+0.001
  Trigonometric Function : Trigonometry
  U1 : Fcn  Expr=u[6]-u[8]
  U2 : Fcn  Expr=u[7]-u[3]
  U3 : Fcn  Expr=u[2]-u[4]
  U_Phi : Fcn  Expr=u[1]+u[5]+u[9]
  U_Phi1 : Fcn  Expr=acos((u(1)-1)/2)
  U_Phi2 : Fcn  Expr=acos((u(1)-1)/2)
  Angles_Visu : Outport
  wires:
  Data Type Conversion/1 -> Mux1/2
  RotMat_Visu/1 -> U1/1, U2/1, U3/1, U_Phi/1
  Trigonometric Function/1 -> Gain/1
  U1/1 -> Mux/1
  U2/1 -> Mux/2
  U3/1 -> Mux/3
  Mux/1 -> Divide/1
  Gain/1 -> Divide/2
  Mux1/1 -> Angles_Visu/1
  Divide/1 -> Mux1/1
  U_Phi/1 -> U_Phi1/1, Saturation1/1
  U_Phi1/1 -> Data Type Conversion/1
  Saturation1/1 -> U_Phi2/1
  U_Phi2/1 -> Trigonometric Function/1

== system V2x_TC_CarBreakdownWarning_cs/VISUWheels_Audi_A8_1/conv_RotWheelRL/RotMat2AxisAngle ==
  RotMat_Visu : Inport
  Data Type Conversion : DataTypeConversion
  Divide : Product  Inputs=*/
  Gain : Gain  Gain=2
  Mux : Mux  Inputs=3
  Mux1 : Mux  Inputs=2
  Saturation1 : Saturate  UpperLimit=3-0.001  LowerLimit=-1+0.001
  Trigonometric Function : Trigonometry
  U1 : Fcn  Expr=u[6]-u[8]
  U2 : Fcn  Expr=u[7]-u[3]
  U3 : Fcn  Expr=u[2]-u[4]
  U_Phi : Fcn  Expr=u[1]+u[5]+u[9]
  U_Phi1 : Fcn  Expr=acos((u(1)-1)/2)
  U_Phi2 : Fcn  Expr=acos((u(1)-1)/2)
  Angles_Visu : Outport
  wires:
  Data Type Conversion/1 -> Mux1/2
  RotMat_Visu/1 -> U1/1, U2/1, U3/1, U_Phi/1
  Trigonometric Function/1 -> Gain/1
  U1/1 -> Mux/1
  U2/1 -> Mux/2
  U3/1 -> Mux/3
  Mux/1 -> Divide/1
  Gain/1 -> Divide/2
  Mux1/1 -> Angles_Visu/1
  Divide/1 -> Mux1/1
  U_Phi/1 -> U_Phi1/1, Saturation1/1
  U_Phi1/1 -> Data Type Conversion/1
  Saturation1/1 -> U_Phi2/1
  U_Phi2/1 -> Trigonometric Function/1

== system V2x_TC_CarBreakdownWarning_cs/VISUWheels_Audi_A8_1/conv_RotWheelRR/RotMat2AxisAngle ==
  RotMat_Visu : Inport
  Data Type Conversion : DataTypeConversion
  Divide : Product  Inputs=*/
  Gain : Gain  Gain=2
  Mux : Mux  Inputs=3
  Mux1 : Mux  Inputs=2
  Saturation1 : Saturate  UpperLimit=3-0.001  LowerLimit=-1+0.001
  Trigonometric Function : Trigonometry
  U1 : Fcn  Expr=u[6]-u[8]
  U2 : Fcn  Expr=u[7]-u[3]
  U3 : Fcn  Expr=u[2]-u[4]
  U_Phi : Fcn  Expr=u[1]+u[5]+u[9]
  U_Phi1 : Fcn  Expr=acos((u(1)-1)/2)
  U_Phi2 : Fcn  Expr=acos((u(1)-1)/2)
  Angles_Visu : Outport
  wires:
  Data Type Conversion/1 -> Mux1/2
  RotMat_Visu/1 -> U1/1, U2/1, U3/1, U_Phi/1
  Trigonometric Function/1 -> Gain/1
  U1/1 -> Mux/1
  U2/1 -> Mux/2
  U3/1 -> Mux/3
  Mux/1 -> Divide/1
  Gain/1 -> Divide/2
  Mux1/1 -> Angles_Visu/1
  Divide/1 -> Mux1/1
  U_Phi/1 -> U_Phi1/1, Saturation1/1
  U_Phi1/1 -> Data Type Conversion/1
  Saturation1/1 -> U_Phi2/1
  U_Phi2/1 -> Trigonometric Function/1

== system V2x_TC_CarBreakdownWarning_cs/VISUWheels_Audi_A8_1/conv_TransWheelFL/pos_ini_Visu ==
  Constant : Constant  Value=x_ini_VRML
  Constant1 : Constant  Value=y_ini_VRML
  Constant2 : Constant  Value=z_ini_VRML
  Mux1 : Mux  Inputs=3
  pos_ini_Visu : Outport
  wires:
  Constant2/1 -> Mux1/3
  Constant1/1 -> Mux1/2
  Mux1/1 -> pos_ini_Visu/1
  Constant/1 -> Mux1/1

== system V2x_TC_CarBreakdownWarning_cs/VISUWheels_Audi_A8_1/conv_TransWheelFL/transISO2Visu ==
  transISO : Inport
  Demux : Demux  Outputs=3
  trans_x_Visu : Outport
  trans_y_Visu : Outport  Port=2
  trans_z_Visu : Outport  Port=3
  wires:
  Demux/3 -> trans_z_Visu/1
  transISO/1 -> Demux/1
  Demux/1 -> trans_x_Visu/1
  Demux/2 -> trans_y_Visu/1  "rot_y"

== system V2x_TC_CarBreakdownWarning_cs/VISUWheels_Audi_A8_1/conv_TransWheelFR/pos_ini_Visu ==
  Constant : Constant  Value=x_ini_VRML
  Constant1 : Constant  Value=y_ini_VRML
  Constant2 : Constant  Value=z_ini_VRML
  Mux1 : Mux  Inputs=3
  pos_ini_Visu : Outport
  wires:
  Constant/1 -> Mux1/1
  Mux1/1 -> pos_ini_Visu/1
  Constant1/1 -> Mux1/2
  Constant2/1 -> Mux1/3

== system V2x_TC_CarBreakdownWarning_cs/VISUWheels_Audi_A8_1/conv_TransWheelFR/transISO2Visu ==
  transISO : Inport
  Demux : Demux  Outputs=3
  trans_x_Visu : Outport
  trans_y_Visu : Outport  Port=2
  trans_z_Visu : Outport  Port=3
  wires:
  Demux/3 -> trans_z_Visu/1
  transISO/1 -> Demux/1
  Demux/1 -> trans_x_Visu/1
  Demux/2 -> trans_y_Visu/1  "rot_y"

== system V2x_TC_CarBreakdownWarning_cs/VISUWheels_Audi_A8_1/conv_TransWheelRL/pos_ini_Visu ==
  Constant : Constant  Value=x_ini_VRML
  Constant1 : Constant  Value=y_ini_VRML
  Constant2 : Constant  Value=z_ini_VRML
  Mux1 : Mux  Inputs=3
  pos_ini_Visu : Outport
  wires:
  Constant/1 -> Mux1/1
  Mux1/1 -> pos_ini_Visu/1
  Constant1/1 -> Mux1/2
  Constant2/1 -> Mux1/3

== system V2x_TC_CarBreakdownWarning_cs/VISUWheels_Audi_A8_1/conv_TransWheelRL/transISO2Visu ==
  transISO : Inport
  Demux : Demux  Outputs=3
  trans_x_Visu : Outport
  trans_y_Visu : Outport  Port=2
  trans_z_Visu : Outport  Port=3
  wires:
  Demux/3 -> trans_z_Visu/1
  transISO/1 -> Demux/1
  Demux/1 -> trans_x_Visu/1
  Demux/2 -> trans_y_Visu/1  "rot_y"

== system V2x_TC_CarBreakdownWarning_cs/VISUWheels_Audi_A8_1/conv_TransWheelRR/pos_ini_Visu ==
  Constant : Constant  Value=x_ini_VRML
  Constant1 : Constant  Value=y_ini_VRML
  Constant2 : Constant  Value=z_ini_VRML
  Mux1 : Mux  Inputs=3
  pos_ini_Visu : Outport
  wires:
  Constant/1 -> Mux1/1
  Mux1/1 -> pos_ini_Visu/1
  Constant1/1 -> Mux1/2
  Constant2/1 -> Mux1/3

== system V2x_TC_CarBreakdownWarning_cs/VISUWheels_Audi_A8_1/conv_TransWheelRR/transISO2Visu ==
  transISO : Inport
  Demux : Demux  Outputs=3
  trans_x_Visu : Outport
  trans_y_Visu : Outport  Port=2
  trans_z_Visu : Outport  Port=3
  wires:
  Demux/3 -> trans_z_Visu/1
  transISO/1 -> Demux/1
  Demux/1 -> trans_x_Visu/1
  Demux/2 -> trans_y_Visu/1  "rot_y"

== system V2x_TC_CarBreakdownWarning_cs/Audi_A8_1/Antenna_Rx_2_Demux/compas converter/cart2compas ==
  Angle [deg] : Inport
  Constant : Constant  Value=90
  Constant1 : Constant  Value=360
  Gain : Gain  Gain=1/360
  Gain1 : Gain  Gain=360
  Gain2 : Gain  Gain=-1
  Rounding Function : Rounding
  Sum : Sum  Inputs=|-+
  Sum1 : Sum  Inputs=-+|
  Sum2 : Sum  Inputs=++|
  heading [deg] : Outport
  wires:
  Gain/1 -> Rounding Function/1
  Rounding Function/1 -> Gain1/1
  Gain1/1 -> Sum/1
  Angle [deg]/1 -> Sum1/2
  Sum/1 -> Gain2/1
  Sum1/1 -> Gain/1, Sum/2
  Constant/1 -> Sum1/1
  Gain2/1 -> Sum2/2
  Constant1/1 -> Sum2/1
  Sum2/1 -> heading [deg]/1

== system V2x_TC_CarBreakdownWarning_cs/Audi_A8_1/Rx_Noise/For Iterator Subsystem1/con1 ==
  tmp_in : Inport
  i : Inport  Port=2
  CAM_in : Inport  Port=3
  Assignment : Assignment  IndexOptions=Index vector (port)  Indices=1  OutputSizes=1
  Bias1 : Bias  Bias=1
  Selector4 : Selector  NumberOfDimensions=2  IndexOptions=Index vector (port),Index vector (dialog)  Indices=[1 3],3  OutputSizes=1,1
  Selector5 : Selector  IndexOptions=Index vector (port)  Indices=[1 3]  OutputSizes=1
  Switch : Switch  Criteria=u2 ~= 0
  tmp_out : Outport
  wires:
  Selector4/1 -> Switch/2
  Assignment/1 -> Switch/1
  Selector5/1 -> Bias1/1
  Bias1/1 -> Assignment/2
  CAM_in/1 -> Selector4/1
  Switch/1 -> tmp_out/1
  tmp_in/1 -> Assignment/1, Selector5/1, Switch/3
  i/1 -> Selector4/2, Assignment/3, Selector5/2

== system V2x_TC_CarBreakdownWarning_cs/Audi_A8_1/Rx_Noise/For Iterator Subsystem1/con2 ==
  CAM_in : Inport
  i : Inport  Port=2
  NoMM : Inport  Port=3
  tmp_in : Inport  Port=4
  Assignment : Assignment  NumberOfDimensions=2  IndexOptions=Index vector (port),Assign all  Indices=1,1  OutputSizes=1,1
  Bias : Bias  Bias=1
  Compare To Zero : simulink/Logic and Bit Operations/Compare To Zero  SystemSampleTime=-1  relop=~=  LogicOutDataTypeMode=boolean
  Compare To Zero1 : simulink/Logic and Bit Operations/Compare To Zero  SystemSampleTime=-1  relop=~=  LogicOutDataTypeMode=boolean
  Constant : Constant  Value=0
  Logical Operator : Logic  AllPortsSameDT=off  OutDataTypeStr=boolean
  Math Function : Math  Operator=mod  SaturateOnIntegerOverflow=on
  Selector4 : Selector  NumberOfDimensions=2  IndexOptions=Index vector (port),Index vector (dialog)  Indices=[1 3],3  OutputSizes=1,1
  Selector5 : Selector  IndexOptions=Index vector (port)  Indices=[1 3]  OutputSizes=1
  Switch : Switch  Criteria=u2 ~= 0
  CAM_o : Outport
  wires:
  Switch/1 -> CAM_o/1
  CAM_in/1 -> Selector4/1, Switch/3, Assignment/1
  Selector4/1 -> Compare To Zero/1
  i/1 -> Selector4/2, Selector5/2, Assignment/3
  Compare To Zero/1 -> Logical Operator/1
  Logical Operator/1 -> Switch/2
  Compare To Zero1/1 -> Logical Operator/2
  Math Function/1 -> Compare To Zero1/1
  tmp_in/1 -> Selector5/1
  Selector5/1 -> Math Function/1
  NoMM/1 -> Bias/1
  Bias/1 -> Math Function/2
  Assignment/1 -> Switch/1
  Constant/1 -> Assignment/2

== system V2x_TC_CarBreakdownWarning_cs/Audi_A8_1/SELF_Demux/compas converter/cart2compas ==
  Angle [deg] : Inport
  Constant : Constant  Value=90
  Constant1 : Constant  Value=360
  Gain : Gain  Gain=1/360
  Gain1 : Gain  Gain=360
  Gain2 : Gain  Gain=-1
  Rounding Function : Rounding
  Sum : Sum  Inputs=|-+
  Sum1 : Sum  Inputs=-+|
  Sum2 : Sum  Inputs=++|
  heading [deg] : Outport
  wires:
  Sum2/1 -> heading [deg]/1
  Constant1/1 -> Sum2/1
  Gain2/1 -> Sum2/2
  Constant/1 -> Sum1/1
  Sum1/1 -> Sum/2, Gain/1
  Sum/1 -> Gain2/1
  Angle [deg]/1 -> Sum1/2
  Gain1/1 -> Sum/1
  Rounding Function/1 -> Gain1/1
  Gain/1 -> Rounding Function/1

== system V2x_TC_CarBreakdownWarning_cs/Audi_A8_1/Traffic Controller/Intersection warning controller/Enabled Subsystem ==
  crossingType : Inport
  hostTurnAdvice : Inport  Port=2
  hostRotZ : Inport  Port=3
  host GPS lat [deg] : Inport  Port=4
  host GPS long [deg] : Inport  Port=5
  host GPS alt [m] : Inport  Port=6
  GPS_lat : Inport  Port=7
  GPS_long : Inport  Port=8
  GPS_alt : Inport  Port=9
  actorID : Inport  Port=10
  targetVelocity : Inport  Port=11
  turnAdvice : Inport  Port=12
  rotZ : Inport  Port=13
  actorType : Inport  Port=14
  crossing detection range : Inport  Port=15
  Enable : EnablePort  PropagateVarSize=During execution
  Intersection : Subsystem
  sort using ID : Subsystem
  warning left lane : Outport
  warning straight lane : Outport  Port=2
  warning right lane : Outport  Port=3
  wires:
  hostRotZ/1 -> Intersection/1(hostRotZ)
  hostTurnAdvice/1 -> Intersection/2(hostTurnAdvice)
  host GPS lat [deg]/1 -> Intersection/3(host GPS lat [deg])
  host GPS long [deg]/1 -> Intersection/4(host GPS long [deg])
  host GPS alt [m]/1 -> Intersection/5(host GPS alt [m])
  actorID/1 -> sort using ID/1(IDs)
  GPS_lat/1 -> sort using ID/2(in1)
  GPS_long/1 -> sort using ID/3(in2)
  GPS_alt/1 -> sort using ID/4(in3)
  targetVelocity/1 -> sort using ID/5(in4)
  turnAdvice/1 -> sort using ID/6(in5)
  rotZ/1 -> sort using ID/7(in6)
  actorType/1 -> sort using ID/8(in7)
  crossingType/1 -> sort using ID/9(in8)
  sort using ID/1(Out1) -> Intersection/6(GPS_lat)
  sort using ID/2(Out2) -> Intersection/7(GPS_long)
  sort using ID/3(Out3) -> Intersection/8(GPS_alt)
  sort using ID/4(Out4) -> Intersection/9(targetVelocity)
  sort using ID/5(Out5) -> Intersection/10(turnAdvice)
  sort using ID/6(Out6) -> Intersection/11(rotZ)
  sort using ID/7(Out7) -> Intersection/12(actorType)
  sort using ID/8(Out8) -> Intersection/13(crossingType)
  Intersection/1(warning left lane) -> warning left lane/1
  Intersection/2(warning straight lane) -> warning straight lane/1
  Intersection/3(warning right lane) -> warning right lane/1
  crossing detection range/1 -> Intersection/14(crossing detection range)

== system V2x_TC_CarBreakdownWarning_cs/Audi_A8_1/Traffic Controller/Road accident detection controller/Compute distance to road accident ==
  conditions : Inport
  host_GPS lat [deg] : Inport  Port=2
  host_GPS lat [deg]1 : Inport  Port=3
  host_GPS alt [m] : Inport  Port=4
  GPS lat [deg] : Inport  Port=5
  GPS long [deg] : Inport  Port=6
  GPS alt [deg] : Inport  Port=7
  Enable : EnablePort  ShowOutputPort=on
  If : If  IfExpression=u1
  If Action Subsystem : Subsystem  TreatAsAtomicUnit=on
  If Action Subsystem1 : Subsystem  TreatAsAtomicUnit=on
  Merge : Merge
  RA_warning : Outport  OutputWhenDisabled=reset  InitialOutput=0
  RA_distance : Outport  Port=2  OutputWhenDisabled=reset  InitialOutput=0
  wires:
  GPS alt [deg]/1 -> If Action Subsystem/4(GPS alt1)
  If/2 -> If Action Subsystem1/Action
  If Action Subsystem1/1(distance) -> Merge/2
  If Action Subsystem/1(distance) -> Merge/1
  GPS long [deg]/1 -> If Action Subsystem/3(GPS long1)
  GPS lat [deg]/1 -> If Action Subsystem/2(GPS lat1)
  If/1 -> If Action Subsystem/Action
  host_GPS lat [deg]1/1 -> If Action Subsystem/6(host_GPS_long)
  host_GPS lat [deg]/1 -> If Action Subsystem/5(host_GPS_lat)
  host_GPS alt [m]/1 -> If Action Subsystem/7(host_GPS_alt)
  Enable/1 -> If/1, RA_warning/1
  conditions/1 -> If Action Subsystem/1(conditions)
  Merge/1 -> RA_distance/1

== system V2x_TC_CarBreakdownWarning_cs/Audi_A8_1/Traffic Controller/Road accident detection controller/distance hold ==
  dist : Inport
  Constant : Constant  Value=0
  Discrete FIR Filter : DiscreteFir  NumCoeffs=0.1 * ones(1,10)
  Memory : Memory
  Switch : Switch  Criteria=u2 > Threshold
  Switch1 : Switch  Criteria=u2 ~= 0
  distance : Outport
  wires:
  dist/1 -> Switch/2, Switch/1, Discrete FIR Filter/1
  Switch/1 -> Memory/1, Switch1/1
  Memory/1 -> Switch/3
  Discrete FIR Filter/1 -> Switch1/2
  Constant/1 -> Switch1/3
  Switch1/1 -> distance/1

== system V2x_TC_CarBreakdownWarning_cs/Audi_A8_1/Traffic Controller/Road accident detection controller/warning hold ==
  warn : Inport
  Constant : Constant  Value=0
  Discrete FIR Filter : DiscreteFir  NumCoeffs=0.1 * ones(1,10)
  Memory : Memory
  Switch : Switch  Criteria=u2 > Threshold
  Switch1 : Switch  Criteria=u2 ~= 0
  warning : Outport
  wires:
  warn/1 -> Switch/2, Switch/1, Discrete FIR Filter/1
  Switch/1 -> Memory/1, Switch1/1
  Memory/1 -> Switch/3
  Discrete FIR Filter/1 -> Switch1/2
  Constant/1 -> Switch1/3
  Switch1/1 -> warning/1
